simulink model "vfod_testing_model"  (R2021b)
settings: Solver=VariableStepAuto  StartTime=0.0  StopTime=30  RelTol=1e-3
libraries: fod x1, vfod_testing x1
settings Model: Creator=Aleksei  LastModifiedBy=Aleksei

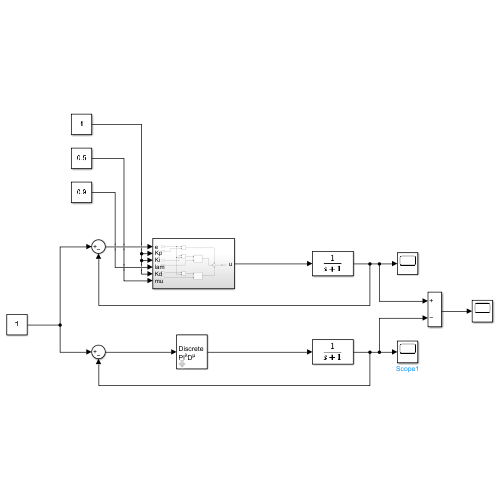
[thumbnail: Simulink's stored preview of the top-level diagram]
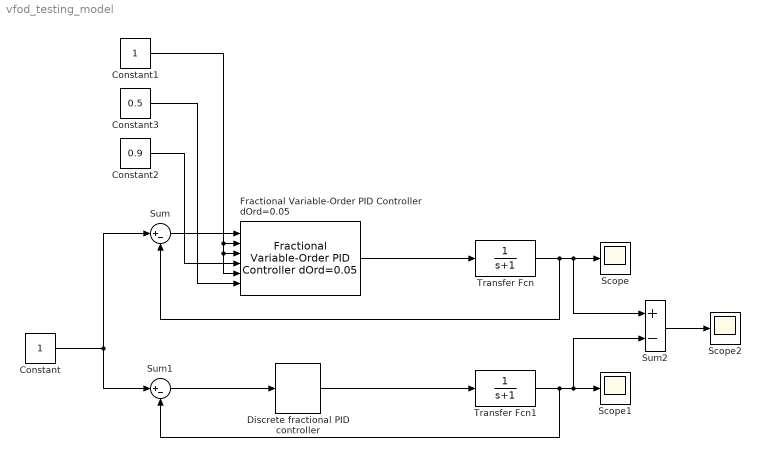
== system vfod_testing_model ==
  Constant : Constant
  Constant1 : Constant
  Constant2 : Constant  Value=0.9
  Constant3 : Constant  Value=0.5
  Discrete fractional PID controller : fod/Discrete fractional PID controller  Kp=1  Ki=1  lambda=0.9  Kd=1  mu=0.5  freqRange=[0.001; 1000]  N=5  useRef=off  dscrMethod=Matched  wc=0  ts=0.01
      settings: SourceProductName=FOMCON Toolbox
  Fractional Variable-Order PID Controller dOrd=0.05 : vfod_testing/Fractional Variable-Order PID Controller dOrd=0.05  SystemSampleTime=-1  VariantActivationTime=update diagram  Latency=0  AutoFrameSizeCalculation=off
  Scope : Scope
  Scope1 : Scope
  Scope2 : Scope
  Sum : Sum  Inputs=|+-
  Sum1 : Sum  Inputs=|+-
  Sum2 : Sum  Inputs=+-
  Transfer Fcn : TransferFcn  Denominator=[1 1]
  Transfer Fcn1 : TransferFcn  Denominator=[1 1]
  wires:
  Fractional Variable-Order PID Controller dOrd=0.05/1 -> Transfer Fcn/1
  Discrete fractional PID controller/1 -> Transfer Fcn1/1
  Sum/1 -> Fractional Variable-Order PID Controller dOrd=0.05/1
  Sum1/1 -> Discrete fractional PID controller/1
  Transfer Fcn/1 -> Sum2/1, Scope/1, Sum/2
  Transfer Fcn1/1 -> Sum2/2, Scope1/1, Sum1/2
  Constant/1 -> Sum1/1, Sum/1
  Constant3/1 -> Fractional Variable-Order PID Controller dOrd=0.05/6
  Constant2/1 -> Fractional Variable-Order PID Controller dOrd=0.05/4
  Constant1/1 -> Fractional Variable-Order PID Controller dOrd=0.05/5, Fractional Variable-Order PID Controller dOrd=0.05/3, Fractional Variable-Order PID Controller dOrd=0.05/2
  Sum2/1 -> Scope2/1
